simulink model "qbot2_sim"  (R2019b)
settings: Solver=FixedStepAuto  StartTime=0.0  StopTime=P.t_end  FixedStep=P.dt  RelTol=1e-3
InitFcn:
  | load_qbot2_sim
StopFcn:
  | plot_sim(out, P)
settings Model: Creator=David L Olson  LastModifiedBy=David L Olson

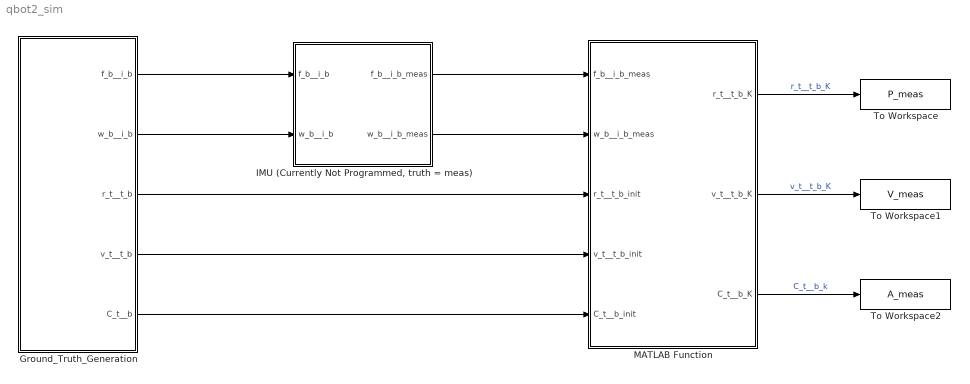
== system qbot2_sim ==
  Ground_Truth_Generation : Subsystem
  "IMU (Currently Not Programmed, truth = meas)" : Subsystem
  MATLAB Function : MATLAB Function  TreatAsAtomicUnit=on
  To Workspace : ToWorkspace  VariableName=P_meas  SaveFormat=Timeseries  SampleTime=-1
  To Workspace1 : ToWorkspace  VariableName=V_meas  SaveFormat=Timeseries  SampleTime=-1
  To Workspace2 : ToWorkspace  VariableName=A_meas  SaveFormat=Timeseries  SampleTime=-1
  wires:
  Ground_Truth_Generation/1(f_b__i_b) -> "IMU (Currently Not Programmed, truth = meas)"/1(f_b__i_b)
  Ground_Truth_Generation/2(w_b__i_b) -> "IMU (Currently Not Programmed, truth = meas)"/2(w_b__i_b)
  "IMU (Currently Not Programmed, truth = meas)"/1(f_b__i_b_meas) -> MATLAB Function/1(f_b__i_b_meas)
  "IMU (Currently Not Programmed, truth = meas)"/2(w_b__i_b_meas) -> MATLAB Function/2(w_b__i_b_meas)
  Ground_Truth_Generation/3(r_t__t_b) -> MATLAB Function/3(r_t__t_b_init)
  Ground_Truth_Generation/4(v_t__t_b) -> MATLAB Function/4(v_t__t_b_init)
  Ground_Truth_Generation/5(C_t__b) -> MATLAB Function/5(C_t__b_init)
  MATLAB Function/1(r_t__t_b_K) -> To Workspace/1  "r_t__t_b_K"
  MATLAB Function/2(v_t__t_b_K) -> To Workspace1/1  "v_t__t_b_K"
  MATLAB Function/3(C_t__b_K) -> To Workspace2/1  "C_t__b_k"

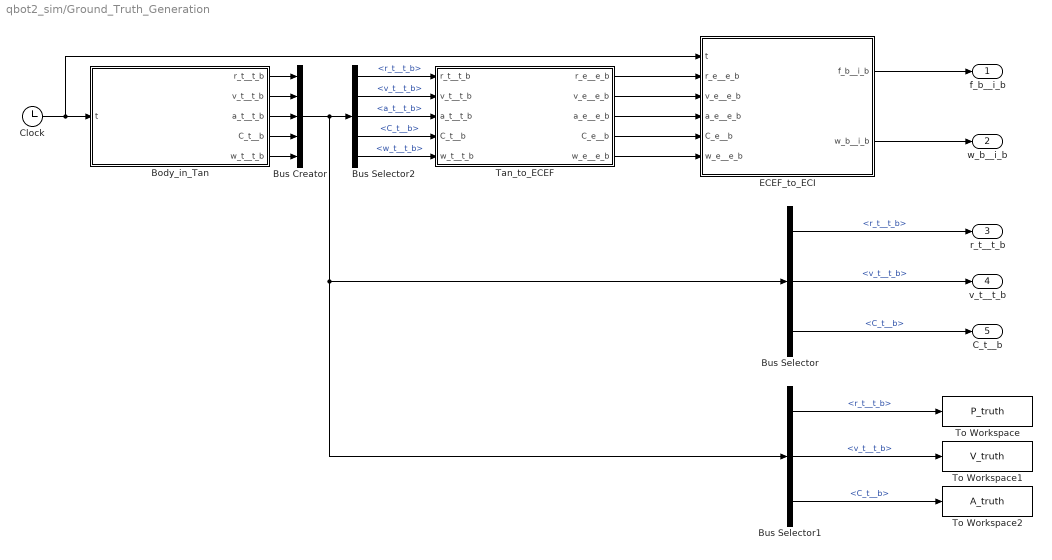
== system qbot2_sim/Ground_Truth_Generation ==
  Body_in_Tan : MATLAB Function  TreatAsAtomicUnit=on
  Bus Creator : BusCreator  Inputs=5
  Bus Selector : BusSelector  OutputSignals=r_t__t_b,v_t__t_b,C_t__b
  Bus Selector1 : BusSelector  OutputSignals=r_t__t_b,v_t__t_b,C_t__b
  Bus Selector2 : BusSelector  OutputSignals=r_t__t_b,v_t__t_b,a_t__t_b,C_t__b,w_t__t_b
  Clock : Clock
  ECEF_to_ECI : MATLAB Function  TreatAsAtomicUnit=on
  Tan_to_ECEF : MATLAB Function  TreatAsAtomicUnit=on
  To Workspace : ToWorkspace  VariableName=P_truth  SaveFormat=Timeseries  SampleTime=-1
  To Workspace1 : ToWorkspace  VariableName=V_truth  SaveFormat=Timeseries  SampleTime=-1
  To Workspace2 : ToWorkspace  VariableName=A_truth  SaveFormat=Timeseries  SampleTime=-1
  f_b__i_b : Outport
  w_b__i_b : Outport  Port=2
  r_t__t_b : Outport  Port=3
  v_t__t_b : Outport  Port=4
  C_t__b : Outport  Port=5
  wires:
  Clock/1 -> Body_in_Tan/1(t), ECEF_to_ECI/1(t)
  Tan_to_ECEF/1(r_e__e_b) -> ECEF_to_ECI/2(r_e__e_b)
  Tan_to_ECEF/3(a_e__e_b) -> ECEF_to_ECI/4(a_e__e_b)
  Tan_to_ECEF/2(v_e__e_b) -> ECEF_to_ECI/3(v_e__e_b)
  Tan_to_ECEF/4(C_e__b) -> ECEF_to_ECI/5(C_e__b)
  Tan_to_ECEF/5(w_e__e_b) -> ECEF_to_ECI/6(w_e__e_b)
  ECEF_to_ECI/2(w_b__i_b) -> w_b__i_b/1
  ECEF_to_ECI/1(f_b__i_b) -> f_b__i_b/1
  Body_in_Tan/1(r_t__t_b) -> Bus Creator/1
  Body_in_Tan/2(v_t__t_b) -> Bus Creator/2
  Body_in_Tan/3(a_t__t_b) -> Bus Creator/3
  Body_in_Tan/4(C_t__b) -> Bus Creator/4
  Body_in_Tan/5(w_t__t_b) -> Bus Creator/5
  Bus Creator/1 -> Bus Selector2/1, Bus Selector/1, Bus Selector1/1
  Bus Selector/1 -> r_t__t_b/1  "<r_t__t_b>"
  Bus Selector/2 -> v_t__t_b/1  "<v_t__t_b>"
  Bus Selector/3 -> C_t__b/1  "<C_t__b>"
  Bus Selector2/5 -> Tan_to_ECEF/5(w_t__t_b)  "<w_t__t_b>"
  Bus Selector2/4 -> Tan_to_ECEF/4(C_t__b)  "<C_t__b>"
  Bus Selector2/3 -> Tan_to_ECEF/3(a_t__t_b)  "<a_t__t_b>"
  Bus Selector2/2 -> Tan_to_ECEF/2(v_t__t_b)  "<v_t__t_b>"
  Bus Selector2/1 -> Tan_to_ECEF/1(r_t__t_b)  "<r_t__t_b>"
  Bus Selector1/2 -> To Workspace1/1  "<v_t__t_b>"
  Bus Selector1/1 -> To Workspace/1  "<r_t__t_b>"
  Bus Selector1/3 -> To Workspace2/1  "<C_t__b>"

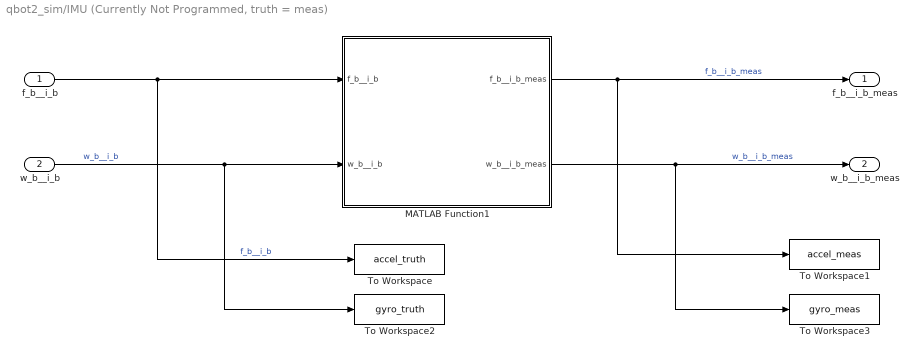
== system qbot2_sim/IMU (Currently Not Programmed, truth = meas) ==
  f_b__i_b : Inport
  w_b__i_b : Inport  Port=2
  MATLAB Function1 : MATLAB Function  TreatAsAtomicUnit=on
  To Workspace : ToWorkspace  VariableName=accel_truth  SaveFormat=Timeseries  SampleTime=-1
  To Workspace1 : ToWorkspace  VariableName=accel_meas  SaveFormat=Timeseries  SampleTime=-1
  To Workspace2 : ToWorkspace  VariableName=gyro_truth  SaveFormat=Timeseries  SampleTime=-1
  To Workspace3 : ToWorkspace  VariableName=gyro_meas  SaveFormat=Timeseries  SampleTime=-1
  f_b__i_b_meas : Outport
  w_b__i_b_meas : Outport  Port=2
  wires:
  f_b__i_b/1 -> To Workspace/1, MATLAB Function1/1(f_b__i_b)  "f_b__i_b"
  w_b__i_b/1 -> To Workspace2/1, MATLAB Function1/2(w_b__i_b)  "w_b__i_b"
  MATLAB Function1/1(f_b__i_b_meas) -> To Workspace1/1, f_b__i_b_meas/1  "f_b__i_b_meas"
  MATLAB Function1/2(w_b__i_b_meas) -> To Workspace3/1, w_b__i_b_meas/1  "w_b__i_b_meas"

== matlab function qbot2_sim/Ground_Truth_Generation/Body_in_Tan ==
  data: r_t__t_b output; v_t__t_b output; a_t__t_b output; C_t__b output; w_t__t_b output; t input; P parameter
function [r_t__t_b, v_t__t_b, a_t__t_b, C_t__b, w_t__t_b] = ...
                                           Body_in_Tan(t, P)
                                       
%% QBOT2_TAN_GROUND_TRUTH_GEN Generates the motion of the body of the Qbot2
%wrt to the tangential frame.  

% Creating figure eight loop pattern for Qbot2.  The motion is unrealistic
% for the robot itself, however for now this verify all equations have been
% implemented correctly in all 3 dimensions.  

persistent init_flag C_t__b_old

% Extra Steps for MATLAB parser to properly function
if (isempty(init_flag))
    init_flag = 0;
    C_t__b_old = eye(3);
end

% Figure Eight Parameters
T = P.t_end;   % Period
f = 1/T;       % Frequency
w = 4*pi*f;    % Natural Frequency

% Figure Eight Amplitudes in {t} frame
Ax = 10;
Ay = 5;
Az = 0.25;

% {t} frame is set Noth East Down (NED)
% Position of {b} wrt {t} in the {t} frame (m) 
r_t__t_b = [      Ax*sin(w*t); ...
                 -Ay*sin((w/2)*t); ...
             Az - Az*cos((2*w)*t)];
        
% Velocity of {b} wrt {t} in the {t} frame (m/s)
v_t__t_b = [    w * Ax*cos(w*t); ...
           -(w/2) * Ay*cos((w/2)*t); ...
            (2*w) * Az*sin((2*w)*t)];
        
% Acceleration of {b} wrt {t} in the {t} frame (m/s^2)
a_t__t_b = [   -w^2 * Ax*sin(w*t); ...
            (w/2)^2 * Ay*sin((w/2)*t); ...
            (2*w)^2 * Az*cos((2*w)*t)];
         
% Orientation of {b} wrt {t} in the {t} frame (forward-right-down frame)
x_axis = v_t__t_b / norm(v_t__t_b); % Due to plant dynamics

% Determine Pitch and Yaw in {t} frame
roll = 0;
pitch = -asin(x_axis(3));
yaw = atan2(x_axis(2), x_axis(1));
C_t__b_temp = ypr2dcm(yaw, pitch, roll);

% Rotate a_t__t_b into {b} frame, compare w/ gravity vector for Roll
a_b__t_b_temp = C_t__b_temp' * a_t__t_b;
roll = atan2(a_b__t_b_temp(2), 10);
C_t__b = ypr2dcm(yaw, pitch, roll); 

if (init_flag == 0) % first time entering function
    w_t__t_b = [0; 0; 0];
    init_flag = 1;
    C_t__b_old = eye(3);
else % Be sure to ask about initial method of what went wrong
    delta_C = C_t__b * C_t__b_old';
    w_t__t_b = dcm2k(delta_C) / P.dt;
end

% Store value of C_t__b for next iteration
C_t__b_old = C_t__b;

end

== matlab function qbot2_sim/MATLAB Function ==
  data: f_b__i_b_meas input; w_b__i_b_meas input; r_t__t_b_init input; v_t__t_b_init input; C_t__b_init input; r_t__t_b_K output; P parameter; v_t__t_b_K output; C_t__b_K output
function [r_t__t_b_K, v_t__t_b_K, C_t__b_K] = Tan_Mech(f_b__i_b_meas, w_b__i_b_meas, r_t__t_b_init, v_t__t_b_init, C_t__b_init, P)

%% Tan_Mech
% Provides tangential mechanization for kinematic states position, velocity
% and attitude (PVA).  It does this solely based on accel and gyro
% measurements, which come from the IMU block.  The first time step is
% initialized from the ground truth block.  

persistent r_t__t_b_K_1 v_t__t_b_K_1 C_t__b_K_1

% Initialize on First Time Step
if (isempty(r_t__t_b_K_1))
    
    % Use "truth" to initialize on first time step
    r_t__t_b_K = r_t__t_b_init;
    v_t__t_b_K = v_t__t_b_init;
    C_t__b_K   = C_t__b_init;
    
    % Store current values as old values for next iteration
    r_t__t_b_K_1 = r_t__t_b_K;
    v_t__t_b_K_1 = v_t__t_b_K;
    C_t__b_K_1   = C_t__b_K;
    
% Every Other Time Step
else
    
    % C_t__b Rotation Matrix Update 
    if (P.fidelity == 0) % Low Fidelity Method
         
        Ohm_b__i_b_meas = vec2ss(w_b__i_b_meas);
        
        C_t__b_K = C_t__b_K_1*(eye(3) + Ohm_b__i_b_meas*P.dt) - ...
                                              P.Ohm_t__i_e*C_t__b_K_1*P.dt;
                                        
    elseif (P.fidelity == 1) % High Fidelity Method
        
        w_t__t_b = C_t__b_K_1*w_b__i_b_meas - P.C_e__t'*P.w_i__i_e;
        
        C_t__b_K = Rodrigues_k(w_t__t_b * P.dt) * C_t__b_K_1;
        
    end
    
    % f_t__i_b Specific Force Update
    f_t__i_b = C_t__b_K * f_b__i_b_meas;
    
    % a_t__t_b Acceleration Vector Update
    r_e__e_b = P.r_e__e_t + P.C_e__t*r_t__t_b_K_1;          % Compute r_e__e_b
    [L_b, lambda_b, h_b] = xyz2llh(r_e__e_b, P);            % Compute the lat, lon, and height
    g_n__b = [0; 0; gravity(L_b, h_b, P)];                  % Compute the acceleration due to gravity
    C_e__n = Lat_Lon_2C_e__n(L_b, lambda_b);                % Compute C_e__n
    g_e__b = C_e__n * g_n__b;                               % Compute the gravity of the body in the {e} frame
    g_t__b = P.C_e__t' * g_e__b;                            % Compute the gravity of the body in the {t} frame 
    a_t__t_b = f_t__i_b + g_t__b - 2*P.Ohm_t__i_e*v_t__t_b_K_1;
    
    % v_t__t_b Velocity Vector Update
    v_t__t_b_K = v_t__t_b_K_1 + a_t__t_b*P.dt;
    
    % r_t__t_b Position Vector Update
    r_t__t_b_K = r_t__t_b_K_1 + v_t__t_b_K_1*P.dt + a_t__t_b*((P.dt^2)/2);
    
    % Store new PVA as old PVA
    r_t__t_b_K_1 = r_t__t_b_K;
    v_t__t_b_K_1 = v_t__t_b_K;
    C_t__b_K_1   = C_t__b_K;
    
end

== matlab function qbot2_sim/Ground_Truth_Generation/Tan_to_ECEF ==
  data: r_t__t_b input; v_t__t_b input; a_t__t_b input; C_t__b input; w_t__t_b input; r_e__e_b output; v_e__e_b output; a_e__e_b output; C_e__b output; w_e__e_b output; P parameter
function [r_e__e_b, v_e__e_b, a_e__e_b, C_e__b, w_e__e_b] = ...
             Tan_to_ECEF(r_t__t_b, v_t__t_b, a_t__t_b, C_t__b, w_t__t_b, P)
         
%% Tan_to_ECEF 
% Transfroms motion in the {t} frame into the {e} frame.  The 'P' structure
% contains data relevant to making the {t}->{e} transforms specifically to
% my house in Minot ND.  (1124 9th St NW, Minot ND 58703)

% Position of the {b} frame wrt the {e} frame resolved in {e} (m)
r_e__e_b = P.r_e__e_t + P.C_e__t*r_t__t_b;

% Velocity of the {b} frame wrt the {e} frame resolved in {e} (m/s)
v_e__e_b = P.C_e__t*v_t__t_b;
       
% Acceleration of the b-frame wrt the e-frame resolved in {e} (m/s^2)
a_e__e_b = P.C_e__t*a_t__t_b;
        
%Attitude of the {b} frame wrt the {e} frame (unitless)
C_e__b = P.C_e__t*C_t__b;         

% Angular velocity of the {b} frame wrt the {e} frame resolved in {e} (rad/s)
w_e__e_b = P.C_e__t*w_t__t_b;

== matlab function qbot2_sim/Ground_Truth_Generation/ECEF_to_ECI ==
  data: t input; f_b__i_b output; r_e__e_b input; v_e__e_b input; a_e__e_b input; C_e__b input; w_e__e_b input; w_b__i_b output; P parameter
function [f_b__i_b, w_b__i_b] = ...
          ECEF_to_ECI(t, r_e__e_b, v_e__e_b, a_e__e_b, C_e__b, w_e__e_b, P)

%% ECEF to ECI
% Transforms motion from the ECEF frame to the ECI frame
% This assumes the simulation always starts at 0000z

% Generate earth's rotation from {i} frame to {e} frame
theta_ie = P.w_ie * t + 0;

C_i__e = [cos(theta_ie), -sin(theta_ie), 0; ...
          sin(theta_ie),  cos(theta_ie), 0; ...
          0,              0,             1];    
      
% Position of {b} frame wrt {t} frame resolved in {i} frame (m)
r_i__i_b = C_i__e*r_e__e_b;

% Velocity of {b} frame wrt {i} frame resolved in {i} frame (m/s)
v_i__i_b = C_i__e*v_e__e_b + P.Ohm_i__i_e*C_i__e*r_e__e_b;

% Acceleration of {b} frame wrt {i} frame resolved in {i} frame (m/s^2)
a_i__i_b = C_i__e*a_e__e_b + 2*P.Ohm_i__i_e*C_i__e*v_e__e_b + ...
                                 P.Ohm_i__i_e*P.Ohm_i__i_e*C_i__e*r_e__e_b;
                                       
% Attitude of {b} frame wrt to {i} frame
C_i__b = C_i__e*C_e__b;

% Angular Velocity: Ideal Gyro Measurements
w_b__i_b = C_i__b' * (P.w_i__i_e + C_i__e*w_e__e_b);

% Specific Force: Ideal Accel Measurements
[L_b, lambda_b, h_b] = xyz2llh(r_e__e_b, P);
g_n__b = [0; 0; gravity(L_b, h_b, P)];
C_e__n = Lat_Lon_2C_e__n(L_b, lambda_b);
g_e__b = C_e__n * g_n__b;
f_b__i_b = C_i__b' * (a_i__i_b - C_i__e*g_e__b - ...
                                       P.Ohm_i__i_e*P.Ohm_i__i_e*r_i__i_b);

== matlab function qbot2_sim/IMU (Currently Not Programmed, truth = meas)/MATLAB Function1 ==
  data: f_b__i_b input; f_b__i_b_meas output; w_b__i_b input; w_b__i_b_meas output; P parameter
function [f_b__i_b_meas, w_b__i_b_meas] = IMU(f_b__i_b, w_b__i_b, P)

% Leaving "Blank" for now...
f_b__i_b_meas = f_b__i_b;
w_b__i_b_meas = w_b__i_b;
